simulink library "FlightSimulation_FlightMechanics_LibModelModified"  (R2023a)
settings: Solver=VariableStepAuto  StartTime=0.0  StopTime=10.0  RelTol=1e-3
undefined symbols (not defined in the file or in its folder): Inertia, mass_lbs
libraries: AeroModel x1, AtmosphericModel x1, EoM_6DoF x1, PropulsionModel x1
settings Model: Creator=LSV-PC0  LastModifiedBy=LSV-PC0

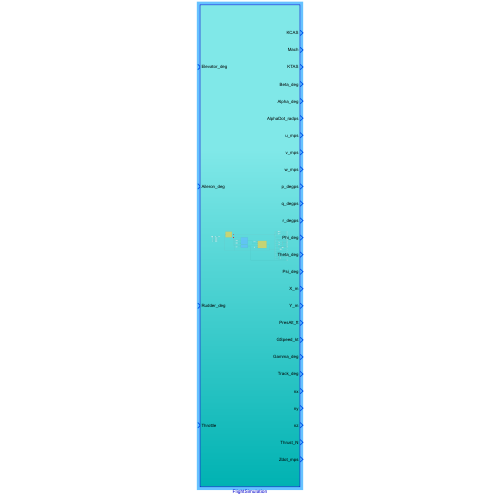
[thumbnail: Simulink's stored preview of the top-level diagram]
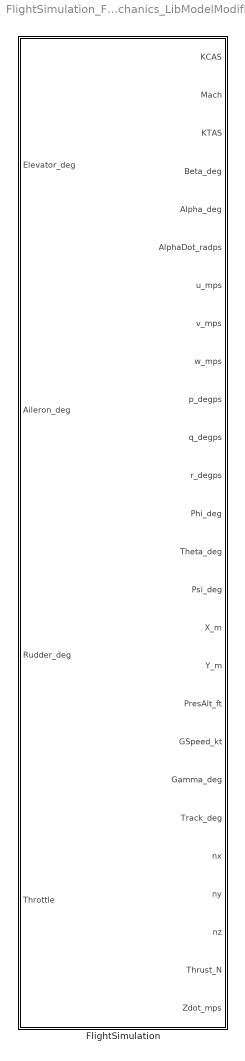
== system FlightSimulation_FlightMechanics_LibModelModified ==
  FlightSimulation : Subsystem

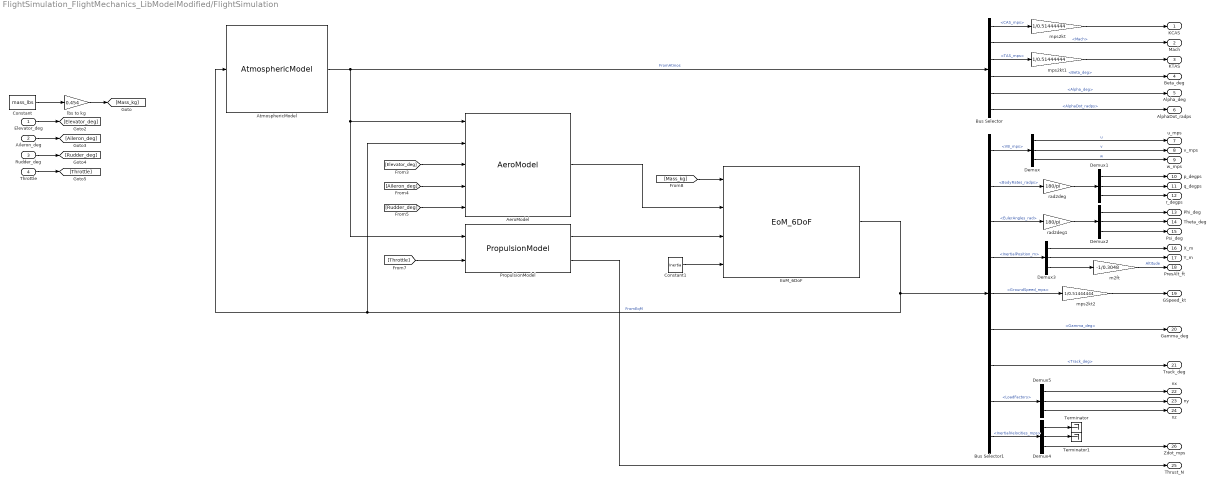
== system FlightSimulation_FlightMechanics_LibModelModified/FlightSimulation ==
  Elevator_deg : Inport  OutDataTypeStr=double
  Aileron_deg : Inport  Port=2  OutDataTypeStr=double
  Rudder_deg : Inport  Port=3  OutDataTypeStr=double
  Throttle : Inport  Port=4  OutDataTypeStr=double
  AeroModel : AeroModel/AeroModel  SystemSampleTime=-1  VariantActivationTime=update diagram  Latency=0  AutoFrameSizeCalculation=off
      link override C_D/Add1: OutMax=[1]
  AtmosphericModel : AtmosphericModel/AtmosphericModel  SystemSampleTime=-1  VariantActivationTime=update diagram  Latency=0  AutoFrameSizeCalculation=off
  Bus Selector : BusSelector  OutputSignals=CAS_mps,Mach,TAS_mps,Beta_deg,Alpha_deg,AlphaDot_radps
  Bus Selector1 : BusSelector  OutputSignals=VB_mps,BodyRates_radps,EulerAngles_rad,InertialPosition_m,GroundSpeed_mps,Gamma_deg,Track_deg,LoadFactors,InertialVelocities_mps
  Constant : Constant  Value=mass_lbs
  Constant1 : Constant  Value=Inertia  OutDataTypeStr=double
  Demux{,1..5} (6 alike) : Demux  Outputs=3
  EoM_6DoF : EoM_6DoF/EoM_6DoF  SystemSampleTime=-1  VariantActivationTime=update diagram  Latency=0  AutoFrameSizeCalculation=off
      link override BodyVelocities/u_mps: InitialCondition=u0
      link override EulerRates/EulerRates/IC: Value=[0 0 0 0 0 0 0 0 0]
      link override EulerRates/PHI_rad: InitialCondition=phi0
      link override EulerRates/PSI_rad: InitialCondition=psi0
      link override EulerRates/THETA_rad: InitialCondition=theta0
      link override InertialData/ZI_m: InitialCondition=Z0
  PropulsionModel : PropulsionModel/PropulsionModel  SystemSampleTime=-1  VariantActivationTime=update diagram  Latency=0  AutoFrameSizeCalculation=off
  Terminator : Terminator
  Terminator1 : Terminator
  lbs to kg : Gain  Gain=0.454
  m2ft : Gain  Gain=-1/0.3048
  mps2kt : Gain  Gain=1/0.51444444
  mps2kt1 : Gain  Gain=1/0.51444444
  mps2kt2 : Gain  Gain=1/0.51444444
  rad2deg : Gain  Gain=180/pi
  rad2deg1 : Gain  Gain=180/pi
  KCAS : Outport
  Mach : Outport  Port=2
  KTAS : Outport  Port=3
  Beta_deg : Outport  Port=4
  Alpha_deg : Outport  Port=5
  AlphaDot_radps : Outport  Port=6
  u_mps : Outport  Port=7
  v_mps : Outport  Port=8
  w_mps : Outport  Port=9
  p_degps : Outport  Port=10
  q_degps : Outport  Port=11
  r_degps : Outport  Port=12
  Phi_deg : Outport  Port=13
  Theta_deg : Outport  Port=14
  Psi_deg : Outport  Port=15
  X_m : Outport  Port=16  OutMax=[1]
  Y_m : Outport  Port=17  OutMax=[1]
  PresAlt_ft : Outport  Port=18  OutMax=[1]
  GSpeed_kt : Outport  Port=19
  Gamma_deg : Outport  Port=20
  Track_deg : Outport  Port=21
  nx : Outport  Port=22
  ny : Outport  Port=23
  nz : Outport  Port=24
  Thrust_N : Outport  Port=25
  Zdot_mps : Outport  Port=26
  wires:
  Demux5/1 -> nx/1
  m2ft/1 -> PresAlt_ft/1  "Altitude"
  Bus Selector1/8 -> Demux5/1  "<LoadFactors>"
  Demux/1 -> u_mps/1  "u"
  Elevator_deg/1 -> [Elevator_deg]
  Demux/3 -> w_mps/1  "w"
  Bus Selector/4 -> Beta_deg/1  "<Beta_deg>"
  Bus Selector/3 -> mps2kt1/1  "<TAS_mps>"
  mps2kt2/1 -> GSpeed_kt/1
  AeroModel/1 -> EoM_6DoF/2
  Demux/2 -> v_mps/1  "v"
  Rudder_deg/1 -> [Rudder_deg]
  Constant/1 -> lbs to kg/1
  AtmosphericModel/1 -> Bus Selector/1, AeroModel/1, PropulsionModel/1  "FromAtmos"
  Aileron_deg/1 -> [Aileron_deg]
  rad2deg1/1 -> Demux2/1
  Bus Selector1/3 -> rad2deg1/1  "<EulerAngles_rad>"
  Throttle/1 -> [Throttle]
  Demux2/1 -> Phi_deg/1
  Demux3/1 -> X_m/1
  Demux2/2 -> Theta_deg/1
  Demux1/1 -> p_degps/1
  [Throttle] -> PropulsionModel/2
  Bus Selector1/6 -> Gamma_deg/1  "<Gamma_deg>"
  [Mass_kg] -> EoM_6DoF/1
  Bus Selector1/2 -> rad2deg/1  "<BodyRates_radps>"
  Constant1/1 -> EoM_6DoF/4
  Bus Selector1/5 -> mps2kt2/1  "<GroundSpeed_mps>"
  PropulsionModel/2 -> Thrust_N/1
  Bus Selector1/4 -> Demux3/1  "<InertialPosition_m>"
  rad2deg/1 -> Demux1/1
  Demux5/3 -> nz/1
  [Aileron_deg] -> AeroModel/4
  Bus Selector/5 -> Alpha_deg/1  "<Alpha_deg>"
  Demux3/3 -> m2ft/1
  Demux1/2 -> q_degps/1
  Demux3/2 -> Y_m/1
  Demux5/2 -> ny/1
  Demux1/3 -> r_degps/1
  [Elevator_deg] -> AeroModel/3
  Bus Selector1/7 -> Track_deg/1  "<Track_deg>"
  PropulsionModel/1 -> EoM_6DoF/3
  mps2kt/1 -> KCAS/1
  [Rudder_deg] -> AeroModel/5
  Bus Selector/2 -> Mach/1  "<Mach>"
  EoM_6DoF/1 -> AtmosphericModel/1, AeroModel/2, Bus Selector1/1  "FromEqM"
  Bus Selector1/1 -> Demux/1  "<VB_mps>"
  Bus Selector/1 -> mps2kt/1  "<CAS_mps>"
  Demux2/3 -> Psi_deg/1
  mps2kt1/1 -> KTAS/1
  Bus Selector/6 -> AlphaDot_radps/1  "<AlphaDot_radps>"
  lbs to kg/1 -> [Mass_kg]
  Bus Selector1/9 -> Demux4/1  "<InertialVelocities_mps>"
  Demux4/1 -> Terminator/1
  Demux4/2 -> Terminator1/1
  Demux4/3 -> Zdot_mps/1
